simulink model "F4_I2C_Master_IWDG"  (R2018b)
settings: Solver=FixedStepDiscrete  StartTime=0.0  StopTime=10.0  FixedStep=0.5  RelTol=1e-3  EnableMultiTasking=on
libraries: I2C_Lib x5, WDG_Lib x1, STM32_Config_Lib x1
settings Model: Creator=liprandd  LastModifiedBy=fenard1
settings DataIOCC: LimitDataPoints=on  SaveFormat=Array  SignalLoggingSaveFormat=ModelDataLogs
settings OptimizationCC: DefaultParameterBehavior=Inlined  DefaultUnderspecifiedDataType=single  InlineInvariantSignals=on  EnhancedBackFolding=on  CachingGlobalReferences=on  PassReuseOutputArgsAs=Individual arguments  LifeSpan=1
settings DebuggingCC: SignalInfNanChecking=error  SolverPrmCheckMsg=warning  UniqueDataStoreMsg=error  AssertControl=DisableAll  AllowSymbolicDim=off  StrictBusMsg=ErrorOnBusTreatedAsVector  SFUnexpectedBacktrackingDiag=warning  SFNoUnconditionalDefaultTransitionDiag=warning  SFUndirectedBroadcastEventsDiag=error  SFExecutionAtInitializationDiag=none
settings HardwareCC: ProdBitPerPointer=32  ProdBitPerSizeT=32  ProdBitPerPtrDiffT=32  ProdLargestAtomicInteger=Integer  ProdWordSize=32  ProdHWDeviceType=STMicroelectronics->STM32 32-bit Cortex-M
settings ModelReferenceCC: PropagateSignalLabelsOutOfModel=off
settings SFSimCC: SimUseLocalCustomCode=off  CompileTimeRecursionLimit=0  EnableRuntimeRecursion=off  MATLABDynamicMemAlloc=off
settings RTWCC: SystemTargetFile=stm32.tlc  TemplateMakefile=stm32.tmf  Description=stm32 (Embedded Target)  GenerateReport=on  RTWUseLocalCustomCode=off
settings CodeAppCC: IgnoreCustomStorageClasses=off  IgnoreTestpoints=on  CustomSymbolStrType=$N$R$M  SimulinkBlockComments=off  StateflowObjectComments=on
settings STFCustomTargetCC: TargetLangStandard=C99 (ISO)  GenerateSampleERTMain=on  ParMdlRefBuildCompliant=on  IncludeMdlTerminateFcn=off  CombineOutputUpdateFcns=on  IncludeFileDelimiter=UseQuote  ERTCustomFileBanners=on  SupportNonFinite=off  SupportComplex=off  SupportContinuousTime=off  SupportNonInlinedSFcns=off  RemoveResetFunc=on  ParenthesesLevel=Maximum  CastingMode=Standards  MATLABClassNameForMDSCustomization=Simulink.SoftwareTarget.ERTCustomization  SystemTargetFile=stm32.tlc
settings ERTTargetCC: TargetLangStandard=C99 (ISO)  MultiwordLength=2048  GenerateSampleERTMain=on  CompOptLevelCompliant=off  ConcurrentExecutionCompliant=off  IncludeMdlTerminateFcn=off  IncludeFileDelimiter=UseQuote  SupportNonFinite=off  SupportComplex=off  ParenthesesLevel=Maximum  CastingMode=Standards  ModelStepFunctionPrototypeControlCompliant=off  CPPClassGenCompliant=off  UseToolchainInfoCompliant=off  ERTSrcFileBannerTemplate=sourceFileTemplate.cgt  ERTHdrFileBannerTemplate=sourceFileTemplate.cgt  ERTDataSrcFileTemplate=sourceFileTemplate.cgt  ERTDataHdrFileTemplate=sourceFileTemplate.cgt  ERTCustomFileTemplate=customRoutineProcess.tlc  ConvertIfToSwitch=off  SuppressUnreachableDefaultCases=off  EnableSignedLeftShifts=off  EnableSignedRightShifts=off
settings ConfigComp: CovMetricSettings=dw  CovHtmlReporting=on  CovSaveCumulativeToWorkspaceVar=on  CovSaveSingleToWorkspaceVar=on  CovExternalEMLEnable=off  CovSFcnEnable=off

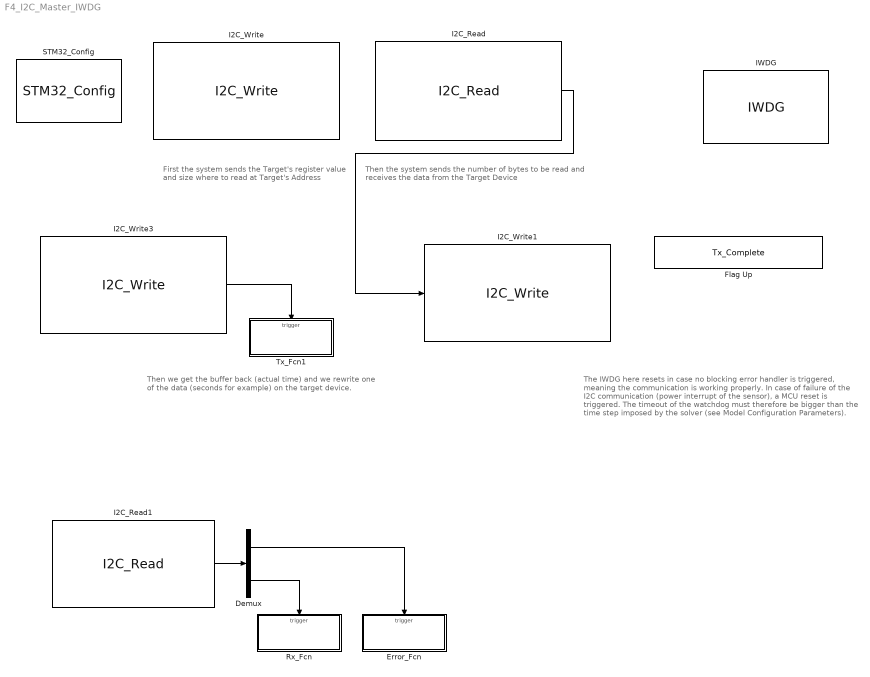
== system F4_I2C_Master_IWDG ==
  note: First the system sends the
      | Target's register value and size
      | where to read at Target's Address
  note: Then the system sends the
      | number of bytes to be read and
      | receives the data from the Target Device
  note: Then we get the buffer back (actual time)
      | and we rewrite one of the data (seconds
      | for example) on the target device.
  note: The IWDG here resets in case no blocking
      | error handler is triggered, meaning the
      | communication is working properly. In case
      | of failure of the I2C communication (power
      | interrupt of the sensor), a MCU reset is triggered.
      | The timeout of the watchdog must therefore be
      | bigger than the time step imposed by the solver
      | (see Model Configuration Parameters).
  Demux : Demux  Outputs=2
  Error_Fcn : Subsystem  TreatAsAtomicUnit=on
  Flag Up : DataStoreMemory  DataStoreName=Tx_Complete  ReadBeforeWriteMsg=warning  WriteAfterWriteMsg=warning  WriteAfterReadMsg=warning  ShowAdditionalParam=off  OutDataTypeStr=boolean
  I2C_Read : I2C_Lib/I2C_Read  Priority=1  i2cx=I2C1  Device_Mode=MASTER  Device_Address=62  i2c_Mode=DMA_RX  Target_Address=0  handler=hi2c1  Buffer_Size=3  Timeout=50  TimeoutValue=25  Enable_Output=on  Error=off  CallBack=off
      settings: SourceProductName=Target Support Package - STM32 Adapter
  I2C_Read1 : I2C_Lib/I2C_Read  i2cx=I2C1  Device_Mode=MASTER  Device_Address=62  i2c_Mode=DMA_RX  Target_Address=0  handler=hi2c1  Buffer_Size=2  Timeout=-1  TimeoutValue=0.5  Enable_Output=off  Error=on  CallBack=on
      settings: SourceProductName=Target Support Package - STM32 Adapter
  I2C_Write : I2C_Lib/I2C_Write  Priority=0  i2cx=I2C1  Device_Mode=MASTER  Target_Address=160  Target_Register=2  Enable_Input=off  Data_str={2}  i2c_Mode=DMA_RX  Buffer_Size=1  handler=hi2c1  Timeout=50  TimeoutValue=25  Error=off  CallBack=off
      settings: SourceProductName=Target Support Package - STM32 Adapter
  I2C_Write1 : I2C_Lib/I2C_Write  Priority=3  i2cx=I2C1  Device_Mode=MASTER  Target_Address=160  Target_Register=2  Enable_Input=on  Data_str_user=0x02,0x44,0x12  Data_str={2,0x02,0x44,0x12}  i2c_Mode=DMA_RX  Buffer_Size=3  handler=hi2c1  Timeout=50  TimeoutValue=25  Error=off  CallBack=off
      settings: SourceProductName=Target Support Package - STM32 Adapter
  I2C_Write3 : I2C_Lib/I2C_Write  Priority=2  i2cx=I2C1  Device_Mode=MASTER  Target_Address=160  Target_Register=2  Enable_Input=off  Data_str={2}  i2c_Mode=DMA_RX  Buffer_Size=1  handler=hi2c1  Timeout=50  TimeoutValue=25  Error=off  CallBack=on
      settings: SourceProductName=Target Support Package - STM32 Adapter
  IWDG : WDG_Lib/IWDG  Reload=7  Custom_Reload=on  Period=56 ms
      settings: SourceProductName=Target Support Package - STM32 Adapter
  Rx_Fcn : Subsystem  TreatAsAtomicUnit=on
  STM32_Config : STM32_Config_Lib/STM32_Config  Project_Path=.\  Config_File=F4_I2C_Master_IWDG.ioc  MCU_Name=STM32F429ZITx
      settings: SourceProductName=Target Support Package - STM32 Adapter
  Tx_Fcn1 : Subsystem  TreatAsAtomicUnit=on
  wires:
  I2C_Read/1 -> I2C_Write1/1
  I2C_Read1/1 -> Demux/1
  Demux/1 -> Error_Fcn/Trigger
  Demux/2 -> Rx_Fcn/Trigger
  I2C_Write3/1 -> Tx_Fcn1/Trigger

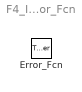
== system F4_I2C_Master_IWDG/Error_Fcn ==
  Error_Fcn : TriggerPort  TriggerType=function-call  VariantControl=Variant

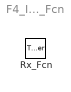
== system F4_I2C_Master_IWDG/Rx_Fcn ==
  Rx_Fcn : TriggerPort  TriggerType=function-call  VariantControl=Variant

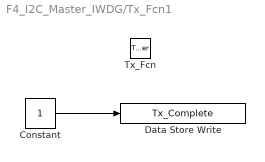
== system F4_I2C_Master_IWDG/Tx_Fcn1 ==
  Tx_Fcn : TriggerPort  TriggerType=function-call  VariantControl=Variant
  Constant : Constant  OutDataTypeStr=boolean
  Data Store Write : DataStoreWrite  DataStoreName=Tx_Complete
  wires:
  Constant/1 -> Data Store Write/1
